simulink model "Estimatoare2021b"  (R2022a)
settings: Solver=VariableStepAuto  StartTime=0.0  StopTime=10  RelTol=1e-3
values from neighbouring files (symbols this model uses):
  AEmd = double(eye(12)+Ts*AE)    [EstimareIntrareNecunoscuta.m]    (also in decuplare.m = double(eye(9)+Ts*Adecup))
  Am = double(round(A(1:9,1:9),4))    [ControllerAroundPointOfOperation.m]    (also in InitializeAircraftPlacePolesCalculateN.m = double(round(A(1:9,1:9),2)); newSys.m)
  Amd = (eye(9)+Ts*Am)    [ControlMinimal.m]    (also in ExtendedControl.m; maimultepuncte.m; newSys.m)
  BEmd = double(Ts*BE)    [EstimareIntrareNecunoscuta.m]    (also in decuplare.m = double(Ts*Bdecup))
  Bm = double(round(B(1:9,1:5),4))    [ControllerAroundPointOfOperation.m]    (also in InitializeAircraftPlacePolesCalculateN.m = double(round(B(1:9,1:5),2)); newSys.m)
  Bmd = Ts*Bm    [ControlMinimal.m]    (also in ExtendedControl.m; maimultepuncte.m; newSys.m)
  CEmd = CE    [EstimareIntrareNecunoscuta.m]    (also in decuplare.m)
  Cm = eye(9)    [newSys.m]
  Cmd = Cm    [ControlMinimal.m]    (also in ExtendedControl.m; maimultepuncte.m; newSys.m)
  F = Ft+Rearth2body(0,Theta,Psi)*Fa+R*G    [aircraftSystem.m]    (also in decuplare.m = T*Adecup-K1*CE; proofCerinteLabEstim.m = T*A-K1*C)
  H = H/z    [ControlMinimal.m]    (also in H.m = [1,tan(Theta)*sin(Phi),tan(Theta)*cos(Phi); decuplare.m = E*pinv(CE*E); proofCerinteLabEstim.m = E*pinv(C*E))
  K = K1+K2    [decuplare.m]
  Km = place(Am,Bm,P)    [ControllerAroundPointOfOperation.m]    (also in InitializeAircraftPlacePolesCalculateN.m; newSys.m)
  Kmd = dlqr(Amd,Bmd,Q,R)    [ControlMinimal.m]    (also in ExtendedControl.m; maimultepuncte.m; newSys.m = lqr(Am-Ld*Cmd,Bm,Q,R))
  L = place(Am',Cm',ObsPoles).'    [newSys.m]
  Ld = place(Amd',Cmd',ObsPoles).'    [newSys.m]
  LEd = place(AEmd',CEmd',ObsPoles).'    [EstimareIntrareNecunoscuta.m]
  pointOfEquilibrium = PointOfEquilibrium(operationStates, operatingInputs ,operatingWinds)    [ControllerAroundPointOfOperation.m]    (also in InitializeAircraftPlacePolesCalculateN.m = PointOfEquilibrium([u0;v0;w0;0;0;0;0;Theta0;Psi0;0;0;100].',; TestMergeFinalLoad.m = PointOfEquilibrium(states,inputs,[-1,-1,-1]); extindere_stari_cu_perturbatie.m = PointOfEquilibrium([u0;0;w0;0;0;0;0;Theta0;Psi0;0;0;100].', ; maimultepuncte.m = GetEquilibriumPoint(UW(i),VW(j),WW(k)))
  T = xinputs(1)    [AMatrixAprox.m]    (also in aircraftSystem.m = u(1); decuplare.m = eye(9)-H*CE; proofCerinteLabEstim.m = eye(3)-H*C)
  Ts = 0.1    [ControlMinimal.m]    (also in EstimareIntrareNecunoscuta.m; ExtendedControl.m; KalmanFilterForExtendedLinearSystem.m; LoadmUltiplePoint.m)
  vant = [1,1,1]*0    [EstimareIntrareNecunoscuta.m]    (also in decuplare.m)
undefined symbols (not defined in the file or in its folder): QExt, RExt
libraries: simulink_extras x7
(part 2 of 2)

== system Estimatoare2021b/estimare intrari necunoscute nu merge bine/system nelinear/perturbatii ==
  Mux1 : Mux  Inputs=3
  Step : Step  Time=0  After=-.1  SampleTime=0
  Step1 : Step  Time=0  After=.1  SampleTime=0
  Step2 : Step  Time=0  After=.1  SampleTime=0
  Out1 : Outport
  wires:
  Step/1 -> Mux1/1
  Step1/1 -> Mux1/2
  Step2/1 -> Mux1/3
  Mux1/1 -> Out1/1

== system Estimatoare2021b/kalman clasic in jurul punctului de echilibru cu controller si zgomot alb pe citire si proces/system nelinear/white noise generator 9x1 ==
  Mux : Mux  Inputs=3
  Random Number : RandomNumber  Variance=.1  SampleTime=Ts
  Random Number1 : RandomNumber  Variance=.1  SampleTime=Ts
  Random Number2 : RandomNumber  Variance=.1  SampleTime=Ts
  d : Outport
  wires:
  Mux/1 -> d/1
  Random Number2/1 -> Mux/3
  Random Number1/1 -> Mux/2
  Random Number/1 -> Mux/1

== system Estimatoare2021b/kalman extins cu controller si zgomot alb pe citire si proces1/kalman extins/Subsystem ==
  states : Inport
  u : Inport  Port=2
  y : Inport  Port=3
  u1 : Inport  Port=4
  Constants : Subsystem
  Memory : Memory  InitialCondition=zeros(9,1)  InheritSampleTime=on
  Memory1 : Memory  InitialCondition=eye(9)*1000
  Zero-Order Hold1 : ZeroOrderHold  SampleTime=Ts
  Zero-Order Hold2 : ZeroOrderHold  SampleTime=Ts
  kalman extins : MATLAB Function  TreatAsAtomicUnit=on
  linearize around poiint of operation : Subsystem
  xest : Outport
  wires:
  Constants/4(Ts) -> kalman extins/10(Ts)
  u1/1 -> kalman extins/11(inputs), linearize around poiint of operation/2(u)
  kalman extins/2(P) -> Memory1/1
  Zero-Order Hold2/1 -> kalman extins/5("P ")
  states/1 -> kalman extins/12(states), linearize around poiint of operation/1(x)
  linearize around poiint of operation/2(B) -> kalman extins/2(Bnew)
  Constants/3(R) -> kalman extins/8(R)
  Constants/2(Cd) -> kalman extins/7(Cd)
  linearize around poiint of operation/1(A) -> kalman extins/1(Anew)
  Memory1/1 -> Zero-Order Hold2/1
  Zero-Order Hold1/1 -> Memory/1
  Constants/1(Q) -> kalman extins/6(Q)
  u/1 -> kalman extins/4(u)
  kalman extins/1(xest) -> Zero-Order Hold1/1
  y/1 -> kalman extins/9(y)
  Memory/1 -> kalman extins/3("xest "), xest/1

== system Estimatoare2021b/kalman extins cu controller si zgomot alb pe citire si proces1/system nelinear/white noise generator 9x1 ==
  Mux : Mux  Inputs=3
  Random Number : RandomNumber  Variance=.1  SampleTime=Ts
  Random Number1 : RandomNumber  Variance=.1  SampleTime=Ts
  Random Number2 : RandomNumber  Variance=.1  SampleTime=Ts
  d : Outport
  wires:
  Mux/1 -> d/1
  Random Number2/1 -> Mux/3
  Random Number1/1 -> Mux/2
  Random Number/1 -> Mux/1

== system Estimatoare2021b/kalman extins cu controller si zgomot alb pe citire si proces1/kalman extins/Subsystem/Constants ==
  Constant1 : Constant  Value=Ts
  Constant2 : Constant  Value=eye(9)
  Constant3 : Constant  Value=QExt
  Constant5 : Constant  Value=RExt
  Q : Outport
  Cd : Outport  Port=2
  R : Outport  Port=3
  Ts : Outport  Port=4
  wires:
  Constant5/1 -> R/1
  Constant3/1 -> Q/1
  Constant2/1 -> Cd/1
  Constant1/1 -> Ts/1

== system Estimatoare2021b/kalman extins cu controller si zgomot alb pe citire si proces1/kalman extins/Subsystem/linearize around poiint of operation ==
  x : Inport
  u : Inport  Port=2
  Interpreted MATLAB Function : MATLABFcn  MATLABFcn=AMatrixAprox  Output1D=off
  Mux : Mux  Inputs=2
  linear operating pioint B matrix : MATLAB Function  TreatAsAtomicUnit=on
  rad2deg : Subsystem
  A : Outport
  B : Outport  Port=2
  wires:
  x/1 -> Mux/2, linear operating pioint B matrix/1(x)
  u/1 -> rad2deg/1(u)
  Interpreted MATLAB Function/1 -> A/1
  linear operating pioint B matrix/1(y) -> B/1
  Mux/1 -> Interpreted MATLAB Function/1
  rad2deg/1(inputs) -> Mux/1, linear operating pioint B matrix/2(inputs)

== system Estimatoare2021b/kalman extins cu controller si zgomot alb pe citire si proces1/kalman extins/Subsystem/linearize around poiint of operation/rad2deg ==
  u : Inport
  Demux : Demux  Outputs=5
  Mux1 : Mux  Inputs=5
  Radians to Degrees{,1..3} (4 alike) : simulink_extras/Transformations/Radians to Degrees
  inputs : Outport
  wires:
  Radians to Degrees1/1 -> Mux1/4
  Radians to Degrees2/1 -> Mux1/3
  Radians to Degrees/1 -> Mux1/5
  Demux/5 -> Radians to Degrees/1
  Demux/3 -> Radians to Degrees2/1
  Demux/4 -> Radians to Degrees1/1
  Demux/1 -> Mux1/1
  u/1 -> Demux/1
  Mux1/1 -> inputs/1
  Radians to Degrees3/1 -> Mux1/2
  Demux/2 -> Radians to Degrees3/1

== matlab function Estimatoare2021b/kalman extins cu controller si zgomot alb pe citire si proces1/kalman extins/Subsystem/linearize around poiint of operation/linear operating pioint B matrix ==
  data: x input; inputs input; y output
function y = jordanB(x,inputs)

%take inputs from vector
T=inputs(1);
DeltaSt=inputs(2);
DeltaRud=inputs(3);
DeltaAlL=inputs(4);
DeltaAlR=inputs(5);
%take states from vector
u=x(1); 
v=x(2);
w=x(3);
p=x(4);
q=x(5);
r=x(6);
Phi=getAngle(x(7));
Theta=getAngle(x(8));
Psi=getAngle(x(9));

y=[100/63,-(540363568592492337*sin(Theta)*(u^2+v^2+w^2))/(4611686018427387904*pi),(63*cos(Theta)*sin(Psi)*(u^2+v^2+w^2))/(2560*pi),-(539*sin(Theta)*(u^2+v^2+w^2))/(16000*pi),-(539*sin(Theta)*(u^2+v^2+w^2))/(16000*pi);
0,0,-(63*cos(Psi)*(u^2+v^2+w^2))/(2560*pi),0,0;
0,-(540363568592492337*cos(Theta)*(u^2+v^2+w^2))/(4611686018427387904*pi),-(63*sin(Psi)*sin(Theta)*(u^2+v^2+w^2))/(2560*pi),-(539*cos(Theta)*(u^2+v^2+w^2))/(16000*pi),-(539*cos(Theta)*(u^2+v^2+w^2))/(16000*pi);
0,0,-(821583*(u^2+v^2+w^2))/(743392000*pi),(250457974518265084593514314168385347*(u^2+v^2+w^2))/(33230699894622896822595176507008614400*pi),-(250457974518265084593514314168385347*(u^2+v^2+w^2))/(33230699894622896822595176507008614400*pi);
0,-(102128714463981051693*(u^2+v^2+w^2))/(2305843009213693952000*pi),0,0,0;
0,0,-(4655637*(u^2+v^2+w^2))/(594713600*pi),(563756479659859815945*(u^2+v^2+w^2))/(1714145246305386374365184*pi),-(563756479659859815945*(u^2+v^2+w^2))/(1714145246305386374365184*pi);
0,0,0,0,0;
0,0,0,0,0;
0,0,0,0,0];
end

== matlab function Estimatoare2021b/estimare intrari necunoscute nu merge bine/system nelinear/MATLAB Function ==
  data: x input; u input; dxdt output; d input
function dxdt = aircraftSystem(x,u,d)
obj=aircraft();
g=9.81;
%take inputs from vector
T=u(1);
DeltaSt=u(2);
DeltaRud=u(3);
DeltaAlL=u(4);
DeltaAlR=u(5);
%take states from vector
u=x(1)-d(1); 
v=x(2)-d(2);
w=x(3)-d(3);
p=x(4);
q=x(5);
r=x(6);
Phi=getAngle(x(7));
Theta=getAngle(x(8));
Psi=getAngle(x(9));
px=x(10);
py=x(11);
pz=x(12);
%vant in earth system
R=Rearth2body(Phi,Theta,Psi);
d=R*d;


alpha=atan2(w,u);
beta=atan2(v,u);
Va2=(u)^2+(v)^2+(w)^2;
Cdw=0.0115*alpha*180/pi+1;
Cdfus=0.075*alpha*180/pi+1;
CyFus=0.075*beta*180/pi;
Cyrud=0.075*(beta+DeltaRud)*180/pi;
Clw=0.11*alpha*180/pi;
ClSt=0.11*(alpha+DeltaSt)*180/pi;
ClwL=0.11*(DeltaAlL+alpha)*180/pi;
ClwR=0.11*(DeltaAlR+alpha)*180/pi;
G=[0;0;obj.m*g];
Fa=[-(Cdw*obj.Af_wing+Cdfus*obj.Af_fuselage)*obj.ro*Va2/2;
-(CyFus*obj.Alat+Cyrud*obj.Arudder)*obj.ro*Va2/2;
-(Clw*obj.Aw+ClSt*obj.Ast+ClwL*obj.Aaileron/2+ClwR*obj.Aaileron/2)*obj.ro*Va2/2];
l_fus=0.01;
Ft=[T;0;0];
% fara vant alpha=theta
% beta=psi
F=Ft+Rearth2body(0,Theta,Psi)*Fa+R*G;

L_bar=obj.l3*obj.Aaileron*(ClwL-ClwR)*obj.ro*Va2/2;
M=(obj.l1*Clw*obj.Aw+ClSt*obj.l2*obj.Ast)*obj.ro*Va2/2;
N=(obj.l2*Cyrud*obj.Arudder+CyFus*l_fus*obj.Alat)*obj.ro*Va2/2;

Moments=[L_bar;M;N];
dxdt=[F/obj.m-cross([p;q;r],[u;v;w]);
    obj.Iinv*(Moments-cross([p;q;r],obj.I*[p;q;r]));
    H(Phi,Theta)*[p;q;r];
    Rbody2earth(-Phi,-Theta,-Psi)*[u;v;w]];
end

== matlab function Estimatoare2021b/decuplare/system nelinear/MATLAB Function ==
  data: x input; u input; dxdt output; d input
function dxdt = aircraftSystem(x,u,d)
obj=aircraft();
g=9.81;
%take inputs from vector
T=u(1);
DeltaSt=u(2);
DeltaRud=u(3);
DeltaAlL=u(4);
DeltaAlR=u(5);
%take states from vector
u=x(1)-d(1); 
v=x(2)-d(2);
w=x(3)-d(3);
p=x(4);
q=x(5);
r=x(6);
Phi=getAngle(x(7));
Theta=getAngle(x(8));
Psi=getAngle(x(9));
px=x(10);
py=x(11);
pz=x(12);
%vant in earth system
R=Rearth2body(Phi,Theta,Psi);
d=R*d;


alpha=atan2(w,u);
beta=atan2(v,u);
Va2=(u)^2+(v)^2+(w)^2;
Cdw=0.0115*alpha*180/pi+1;
Cdfus=0.075*alpha*180/pi+1;
CyFus=0.075*beta*180/pi;
Cyrud=0.075*(beta+DeltaRud)*180/pi;
Clw=0.11*alpha*180/pi;
ClSt=0.11*(alpha+DeltaSt)*180/pi;
ClwL=0.11*(DeltaAlL+alpha)*180/pi;
ClwR=0.11*(DeltaAlR+alpha)*180/pi;
G=[0;0;obj.m*g];
Fa=[-(Cdw*obj.Af_wing+Cdfus*obj.Af_fuselage)*obj.ro*Va2/2;
-(CyFus*obj.Alat+Cyrud*obj.Arudder)*obj.ro*Va2/2;
-(Clw*obj.Aw+ClSt*obj.Ast+ClwL*obj.Aaileron/2+ClwR*obj.Aaileron/2)*obj.ro*Va2/2];
l_fus=0.01;
Ft=[T;0;0];
% fara vant alpha=theta
% beta=psi
F=Ft+Rearth2body(0,Theta,Psi)*Fa+R*G;

L_bar=obj.l3*obj.Aaileron*(ClwL-ClwR)*obj.ro*Va2/2;
M=(obj.l1*Clw*obj.Aw+ClSt*obj.l2*obj.Ast)*obj.ro*Va2/2;
N=(obj.l2*Cyrud*obj.Arudder+CyFus*l_fus*obj.Alat)*obj.ro*Va2/2;

Moments=[L_bar;M;N];
dxdt=[F/obj.m-cross([p;q;r],[u;v;w]);
    obj.Iinv*(Moments-cross([p;q;r],obj.I*[p;q;r]));
    H(Phi,Theta)*[p;q;r];
    Rbody2earth(-Phi,-Theta,-Psi)*[u;v;w]];
end

== matlab function Estimatoare2021b/System neliniar cu controller si estimator total/system nelinear/MATLAB Function ==
  data: x input; u input; dxdt output; d input
function dxdt = aircraftSystem(x,u,d)
obj=aircraft();
g=9.81;
%take inputs from vector
T=u(1);
DeltaSt=getAngle(u(2));
DeltaRud=getAngle(u(3));
DeltaAlL=getAngle(u(4));
DeltaAlR=getAngle(u(5));
%take states from vector
u=x(1)-d(1); 
v=x(2)-d(2);
w=x(3)-d(3);
p=x(4);
q=x(5);
r=x(6);
Phi=getAngle(x(7));
Theta=getAngle(x(8));
Psi=getAngle(x(9));
px=x(10);
py=x(11);
pz=x(12);
%vant in earth system
R=Rearth2body(Phi,Theta,Psi);
d=R*d;


alpha=atan2(w,u);
beta=atan2(v,u);
Va2=(u)^2+(v)^2+(w)^2;
Cdw=0.0115*alpha*180/pi+1;
Cdfus=0.075*alpha*180/pi+1;
CyFus=0.075*beta*180/pi;
Cyrud=0.075*(beta+DeltaRud)*180/pi;
Clw=0.11*alpha*180/pi;
ClSt=0.11*(alpha+DeltaSt)*180/pi;
ClwL=0.11*(DeltaAlL+alpha)*180/pi;
ClwR=0.11*(DeltaAlR+alpha)*180/pi;
G=[0;0;obj.m*g];
Fa=[-(Cdw*obj.Af_wing+Cdfus*obj.Af_fuselage)*obj.ro*Va2/2;
-(CyFus*obj.Alat+Cyrud*obj.Arudder)*obj.ro*Va2/2;
-(Clw*obj.Aw+ClSt*obj.Ast+ClwL*obj.Aaileron/2+ClwR*obj.Aaileron/2)*obj.ro*Va2/2];
l_fus=0.01;
Ft=[T;0;0];
% fara vant alpha=theta
% beta=psi
F=Ft+Rearth2body(0,Theta,Psi)*Fa+R*G;

L_bar=obj.l3*obj.Aaileron*(ClwL-ClwR)*obj.ro*Va2/2;
M=(obj.l1*Clw*obj.Aw+ClSt*obj.l2*obj.Ast)*obj.ro*Va2/2;
N=(obj.l2*Cyrud*obj.Arudder+CyFus*l_fus*obj.Alat)*obj.ro*Va2/2;

Moments=[L_bar;M;N];
dxdt=[F/obj.m-cross([p;q;r],[u;v;w]);
    obj.Iinv*(Moments-cross([p;q;r],obj.I*[p;q;r]));
    H(Phi,Theta)*[p;q;r];
    Rbody2earth(-Phi,-Theta,-Psi)*[u;v;w]];
end

== matlab function Estimatoare2021b/System neliniar in 0 cu intrari 0/MATLAB Function ==
  data: x input; u input; dxdt output; d input
function dxdt = aircraftSystem(x,u,d)
obj=aircraft();
g=9.81;
%take inputs from vector
T=u(1);
DeltaSt=u(2);
DeltaRud=u(3);
DeltaAlL=u(4);
DeltaAlR=u(5);
%take states from vector
u=x(1)-d(1); 
v=x(2)-d(2);
w=x(3)-d(3);
p=x(4);
q=x(5);
r=x(6);
Phi=getAngle(x(7));
Theta=getAngle(x(8));
Psi=getAngle(x(9));
px=x(10);
py=x(11);
pz=x(12);
%vant in earth system
R=Rearth2body(Phi,Theta,Psi);
d=R*d;


alpha=atan2(w,u);
beta=atan2(v,u);
Va2=(u)^2+(v)^2+(w)^2;
Cdw=0.0115*alpha*180/pi+1;
Cdfus=0.075*alpha*180/pi+1;
CyFus=0.075*beta*180/pi;
Cyrud=0.075*(beta+DeltaRud)*180/pi;
Clw=0.11*alpha*180/pi;
ClSt=0.11*(alpha+DeltaSt)*180/pi;
ClwL=0.11*(DeltaAlL+alpha)*180/pi;
ClwR=0.11*(DeltaAlR+alpha)*180/pi;
G=[0;0;obj.m*g];
Fa=[-(Cdw*obj.Af_wing+Cdfus*obj.Af_fuselage)*obj.ro*Va2/2;
-(CyFus*obj.Alat+Cyrud*obj.Arudder)*obj.ro*Va2/2;
-(Clw*obj.Aw+ClSt*obj.Ast+ClwL*obj.Aaileron/2+ClwR*obj.Aaileron/2)*obj.ro*Va2/2];
l_fus=0.01;
Ft=[T;0;0];
% fara vant alpha=theta
% beta=psi
Fa=[0;0;0];
F=Ft+Rearth2body(0,Theta,Psi)*Fa+R*G;

L_bar=obj.l3*obj.Aaileron*(ClwL-ClwR)*obj.ro*Va2/2;
M=(obj.l1*Clw*obj.Aw+ClSt*obj.l2*obj.Ast)*obj.ro*Va2/2;
N=(obj.l2*Cyrud*obj.Arudder+CyFus*l_fus*obj.Alat)*obj.ro*Va2/2;

Moments=[0;0;0];

dxdt=[F/obj.m-cross([p;q;r],[u;v;w]);
    obj.Iinv*(Moments-cross([p;q;r],obj.I*[p;q;r]));
    H(alpha,beta)*[p;q;r];
    Rbody2earth(-Phi,-Theta,-Psi)*[u;v;w]];
end

== matlab function Estimatoare2021b/estimator in timp discret si controller discret pe model nelinear/system nelinear/MATLAB Function ==
  data: x input; u input; dxdt output; d input
function dxdt = aircraftSystem(x,u,d)
obj=aircraft();
g=9.81;
%take inputs from vector
T=u(1);
DeltaSt=getAngle(u(2));
DeltaRud=getAngle(u(3));
DeltaAlL=getAngle(u(4));
DeltaAlR=getAngle(u(5));
%take states from vector
u=x(1)-d(1); 
v=x(2)-d(2);
w=x(3)-d(3);
p=x(4);
q=x(5);
r=x(6);
Phi=getAngle(x(7));
Theta=getAngle(x(8));
Psi=getAngle(x(9));
px=x(10);
py=x(11);
pz=x(12);
%vant in earth system
R=Rearth2body(Phi,Theta,Psi);
d=R*d;


alpha=atan2(w,u);
beta=atan2(v,u);
Va2=(u)^2+(v)^2+(w)^2;
Cdw=0.0115*alpha*180/pi+1;
Cdfus=0.075*alpha*180/pi+1;
CyFus=0.075*beta*180/pi;
Cyrud=0.075*(beta+DeltaRud)*180/pi;
Clw=0.11*alpha*180/pi;
ClSt=0.11*(alpha+DeltaSt)*180/pi;
ClwL=0.11*(DeltaAlL+alpha)*180/pi;
ClwR=0.11*(DeltaAlR+alpha)*180/pi;
G=[0;0;obj.m*g];
Fa=[-(Cdw*obj.Af_wing+Cdfus*obj.Af_fuselage)*obj.ro*Va2/2;
-(CyFus*obj.Alat+Cyrud*obj.Arudder)*obj.ro*Va2/2;
-(Clw*obj.Aw+ClSt*obj.Ast+ClwL*obj.Aaileron/2+ClwR*obj.Aaileron/2)*obj.ro*Va2/2];
l_fus=0.01;
Ft=[T;0;0];
% fara vant alpha=theta
% beta=psi
F=Ft+Rearth2body(0,Theta,Psi)*Fa+R*G;

L_bar=obj.l3*obj.Aaileron*(ClwL-ClwR)*obj.ro*Va2/2;
M=(obj.l1*Clw*obj.Aw+ClSt*obj.l2*obj.Ast)*obj.ro*Va2/2;
N=(obj.l2*Cyrud*obj.Arudder+CyFus*l_fus*obj.Alat)*obj.ro*Va2/2;

Moments=[L_bar;M;N];
dxdt=[F/obj.m-cross([p;q;r],[u;v;w]);
    obj.Iinv*(Moments-cross([p;q;r],obj.I*[p;q;r]));
    H(Phi,Theta)*[p;q;r];
    Rbody2earth(-Phi,-Theta,-Psi)*[u;v;w]];
end

== matlab function Estimatoare2021b/kalman clasic in jurul punctului de echilibru cu controller si zgomot alb pe citire si proces/system nelinear/MATLAB Function ==
  data: x input; u input; dxdt output; d input
function dxdt = aircraftSystem(x,u,d)
obj=aircraft();
g=9.81;
%take inputs from vector
T=u(1);
DeltaSt=getAngle(u(2));
DeltaRud=getAngle(u(3));
DeltaAlL=getAngle(u(4));
DeltaAlR=getAngle(u(5));
%take states from vector
u=x(1)-d(1); 
v=x(2)-d(2);
w=x(3)-d(3);
p=x(4);
q=x(5);
r=x(6);
Phi=getAngle(x(7));
Theta=getAngle(x(8));
Psi=getAngle(x(9));
px=x(10);
py=x(11);
pz=x(12);
%vant in earth system
R=Rearth2body(Phi,Theta,Psi);
d=R*d;


alpha=atan2(w,u);
beta=atan2(v,u);
Va2=(u)^2+(v)^2+(w)^2;
Cdw=0.0115*alpha*180/pi+1;
Cdfus=0.075*alpha*180/pi+1;
CyFus=0.075*beta*180/pi;
Cyrud=0.075*(beta+DeltaRud)*180/pi;
Clw=0.11*alpha*180/pi;
ClSt=0.11*(alpha+DeltaSt)*180/pi;
ClwL=0.11*(DeltaAlL+alpha)*180/pi;
ClwR=0.11*(DeltaAlR+alpha)*180/pi;
G=[0;0;obj.m*g];
Fa=[-(Cdw*obj.Af_wing+Cdfus*obj.Af_fuselage)*obj.ro*Va2/2;
-(CyFus*obj.Alat+Cyrud*obj.Arudder)*obj.ro*Va2/2;
-(Clw*obj.Aw+ClSt*obj.Ast+ClwL*obj.Aaileron/2+ClwR*obj.Aaileron/2)*obj.ro*Va2/2];
l_fus=0.01;
Ft=[T;0;0];
% fara vant alpha=theta
% beta=psi
F=Ft+Rearth2body(0,Theta,Psi)*Fa+R*G;

L_bar=obj.l3*obj.Aaileron*(ClwL-ClwR)*obj.ro*Va2/2;
M=(obj.l1*Clw*obj.Aw+ClSt*obj.l2*obj.Ast)*obj.ro*Va2/2;
N=(obj.l2*Cyrud*obj.Arudder+CyFus*l_fus*obj.Alat)*obj.ro*Va2/2;

Moments=[L_bar;M;N];
dxdt=[F/obj.m-cross([p;q;r],[u;v;w]);
    obj.Iinv*(Moments-cross([p;q;r],obj.I*[p;q;r]));
    H(Phi,Theta)*[p;q;r];
    Rbody2earth(-Phi,-Theta,-Psi)*[u;v;w]];
end

== matlab function Estimatoare2021b/kalman clasic in jurul punctului de echilibru cu controller si zgomot alb pe citire si proces/kalman/MATLAB Function ==
  data: Ad input; Bd input; xest output; y input; Cd input; xpred input; u input; P input; P output; Q input; R input
function [xest,P] = KalmanFilterNoCap(Ad, Bd, y, Cd, xpred, u, P, Q, R)
    xpred=Ad*xpred+Bd*u;
    Pred=Ad*P*Ad.'+Q;
    Kn=Pred*Cd.'/(Cd*Pred*Cd.'+R);
    xest=xpred+Kn*(y-Cd*xpred);
    P=(eye(9)-Kn*Cd)*Pred*(eye(9)-Kn*Cd).'+Kn*R*Kn.';
end

== matlab function Estimatoare2021b/kalman extins cu controller si zgomot alb pe citire si proces1/kalman extins/Subsystem/kalman extins ==
  data: Anew input; Bnew input; xest input; u input; P input; Q input; Cd input; R input; y input; Ts input; inputs input; states input; xest output; P output
function [xest,P] = KalmanFilterExtendedCox(Anew,Bnew, xest, u, P, Q, Cd, R, y,Ts,inputs,states)
   
    %liniarizam in jurul noilui punct de echilibri
    Ad=eye(9)+Ts*double(Anew);
    Bd=Ts*double(Bnew);
    %facem predictie
    xpred=Ad*(xest)+Bd*(u-inputs);
    %recaluculam greutatea predictiei
    Pred=Ad*P*Ad.'+Q;
    %recalculam castig kalman
    Kn=Pred*Cd.'/(Cd*Pred*Cd.'+R);
    %facem estimare
    xest=xpred+Kn*(y-Cd*(xpred+states));
    %actualizam P
    P=(eye(9)-Kn*Cd)*Pred*(eye(9)-Kn*Cd).'+Kn*R*Kn.';
end

== matlab function Estimatoare2021b/kalman extins cu controller si zgomot alb pe citire si proces1/system nelinear/MATLAB Function ==
  data: x input; u input; dxdt output; d input
function dxdt = aircraftSystem(x,u,d)
obj=aircraft();
g=9.81;
%take inputs from vector
T=u(1);
DeltaSt=getAngle(u(2));
DeltaRud=getAngle(u(3));
DeltaAlL=getAngle(u(4));
DeltaAlR=getAngle(u(5));
%take states from vector
u=x(1)-d(1); 
v=x(2)-d(2);
w=x(3)-d(3);
p=x(4);
q=x(5);
r=x(6);
Phi=getAngle(x(7));
Theta=getAngle(x(8));
Psi=getAngle(x(9));
px=x(10);
py=x(11);
pz=x(12);
%vant in earth system
R=Rearth2body(Phi,Theta,Psi);
d=R*d;


alpha=atan2(w,u);
beta=atan2(v,u);
Va2=(u)^2+(v)^2+(w)^2;
Cdw=0.0115*alpha*180/pi+1;
Cdfus=0.075*alpha*180/pi+1;
CyFus=0.075*beta*180/pi;
Cyrud=0.075*(beta+DeltaRud)*180/pi;
Clw=0.11*alpha*180/pi;
ClSt=0.11*(alpha+DeltaSt)*180/pi;
ClwL=0.11*(DeltaAlL+alpha)*180/pi;
ClwR=0.11*(DeltaAlR+alpha)*180/pi;
G=[0;0;obj.m*g];
Fa=[-(Cdw*obj.Af_wing+Cdfus*obj.Af_fuselage)*obj.ro*Va2/2;
-(CyFus*obj.Alat+Cyrud*obj.Arudder)*obj.ro*Va2/2;
-(Clw*obj.Aw+ClSt*obj.Ast+ClwL*obj.Aaileron/2+ClwR*obj.Aaileron/2)*obj.ro*Va2/2];
l_fus=0.01;
Ft=[T;0;0];
% fara vant alpha=theta
% beta=psi
F=Ft+Rearth2body(0,Theta,Psi)*Fa+R*G;

L_bar=obj.l3*obj.Aaileron*(ClwL-ClwR)*obj.ro*Va2/2;
M=(obj.l1*Clw*obj.Aw+ClSt*obj.l2*obj.Ast)*obj.ro*Va2/2;
N=(obj.l2*Cyrud*obj.Arudder+CyFus*l_fus*obj.Alat)*obj.ro*Va2/2;

Moments=[L_bar;M;N];
dxdt=[F/obj.m-cross([p;q;r],[u;v;w]);
    obj.Iinv*(Moments-cross([p;q;r],obj.I*[p;q;r]));
    H(Phi,Theta)*[p;q;r];
    Rbody2earth(-Phi,-Theta,-Psi)*[u;v;w]];
end
